simulink model "sim_elicottero"  (R2025b)
settings: Solver=VariableStepAuto  StartTime=0.0  StopTime=200  RelTol=1e-3
values from neighbouring files (symbols this model uses):
  A_nom = double(subs(A_sym_nom, [x;u], [x0;u0]))    [dataset_elicottero.m]
  aero = evalin('base','aero')    [analisi_LQG.m]
  alpha_0 = deg2rad(10)    [dataset_elicottero.m]
  B_ext_nom = [B_nom Bd_nom]    [dataset_elicottero.m]
  beta_0 = 0    [dataset_elicottero.m]
  C_angles = [ ... (first row only)    [actuator_lumped_uncertainty.m]    (also in analisi_montecarlo.m = [1 0 0 0; 0 0 1 0]; dataset_elicottero.m)
  Ddec_phys = [8.48868560985e-05  4.80771131122e-11; -3.04359895869e-06  1.06562367592e-06]    [HINF_controllers.mat]    (also in Hinf_hinfstruct.m = Du *      Ddec_scaled *      Du_inv; Hinf_synthesis_full.m = Du *      Ddec_scaled *      inv(Du))
  den_2nd = [1, 2*zeta*omega_n, omega_n^2]    [dataset_elicottero.m]
  denFalpha = [1 24.6158182311]    [HINF_controllers.mat]
  denFbeta = [1 13.1899797029]    [HINF_controllers.mat]
  F1_0 = u0_nom(1)    [dataset_elicottero.m]
  F2_0 = u0_nom(2)    [dataset_elicottero.m]
  HalphaBeta = (C_angle_meas.'*Vinv*C_angle_meas) \      (C_angle_meas.'*Vinv)    [dataset_elicottero.m]
  K_hinfsyn = minreal(          Du *          K_hinfsyn_scaled *          Dy_inv,          1e-7)    [Hinf_hinfstruct.m]    (also in Hinf_synthesis_full.m = minreal(          Du *          K_hinfsyn_scaled *          )
  K_lqg_2dof = ss(      Ac_ctrl,      Bc_ctrl,      Cc_ctrl,      Dc_ctrl)    [LQG_reg_2DOF.m]
  K_lqg_int = ss(      Ac_ctrl,      [Bcr Bcy],      Cc_ctrl,      Dc_ctrl)    [LQG_con_integratore.m]
  K_mix = minreal(          Du *          K_mix_scaled *          Dy_inv,          1e-7)    [Hinf_hinfstruct.m]    (also in Hinf_synthesis_full.m = minreal(          Du *          K_mix_scaled *          Dy_i)
  K_mu = Du * K_mu_scaled * Dy_inv    [mu_synthesis.m]
  Kalpha_tuned = pid(          alphaScaledToPhys *          Kalpha_tuned_scaled.Kp,          alphaScaledToPhys *          Kalpha_tuned_scaled.Ki,          alphaScaledToPhys *          Kalpha_tuned_scaled.Kd,          Kalpha_tuned_scaled.Tf)    [Hinf_hinfstruct.m]    (also in Hinf_synthesis_full.m = pid(          alphaScaledToPhys * Kalpha_tuned_scaled.Kp,   )
  Kbeta_tuned = pid(          betaScaledToPhys *          Kbeta_tuned_scaled.Kp,          betaScaledToPhys *          Kbeta_tuned_scaled.Ki,          betaScaledToPhys *          Kbeta_tuned_scaled.Kd,          Kbeta_tuned_scaled.Tf)    [Hinf_hinfstruct.m]    (also in Hinf_synthesis_full.m = pid(          betaScaledToPhys * Kbeta_tuned_scaled.Kp,     )
  mx_eq = cos(alpha_0) * cos(beta_0)    [dataset_elicottero.m]
  my_eq = -sin(beta_0)    [dataset_elicottero.m]
  num_2nd = omega_n^2    (= 900)    [dataset_elicottero.m]
  numFalpha = [16.7939294955 590.000844903]    [HINF_controllers.mat]
  numFbeta = [34.4835250476 9.60244651319]    [HINF_controllers.mat]
  P_nom_ext = ss(      A_nom,      B_ext_nom,      Cy,      zeros(3,4))    [dataset_elicottero.m]
  tau_d_nom = 0.02    [dataset_elicottero.m]
  umax = 5    [LQG_con_integratore.m]    (also in LQG_reg_1DOF.m; analisi_montecarlo.m = 2.5; dataset_elicottero.m)
  y_acc_eq = -p.g * sin(alpha_0)    [dataset_elicottero.m]
undefined symbols (not defined in the file or in its folder): act, sensor
libraries: simulink x20, slpidlib x2, cstblocks x2
(part 1 of 2)
settings Model: Creator=LUCA  LastModifiedBy=39345
settings DataIOCC: SaveState=on  StateSaveName=xhat_out

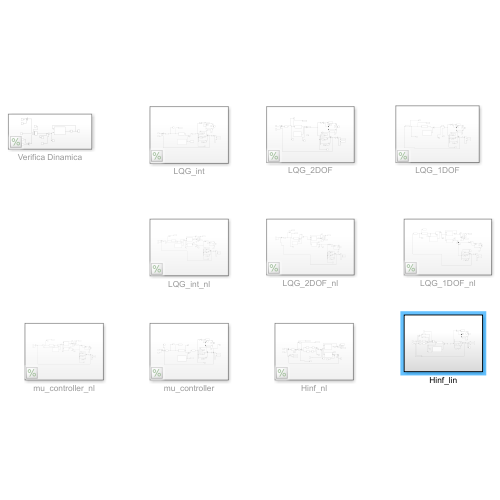
[thumbnail: Simulink's stored preview of the top-level diagram]
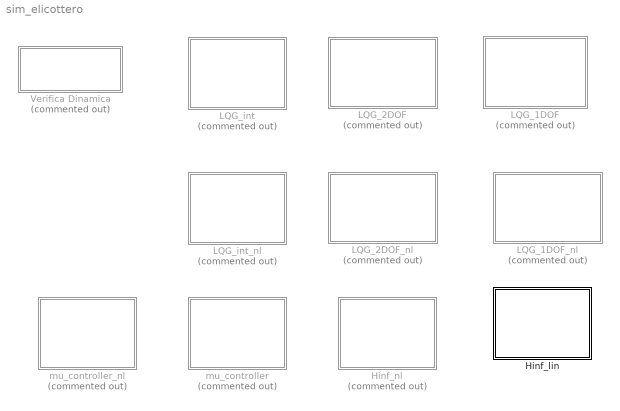
== system sim_elicottero ==
  Hinf_lin : Subsystem
  Hinf_nl : Subsystem  Commented=on
  LQG_1DOF : Subsystem  Commented=on
  LQG_1DOF_nl : Subsystem  Commented=on
  LQG_2DOF : Subsystem  Commented=on
  LQG_2DOF_nl : Subsystem  Commented=on
  LQG_int : Subsystem  Commented=on
  LQG_int_nl : Subsystem  Commented=on
  Verifica Dinamica : Subsystem  Commented=on
  mu_controller : Subsystem  Commented=on
  mu_controller_nl : Subsystem  Commented=on

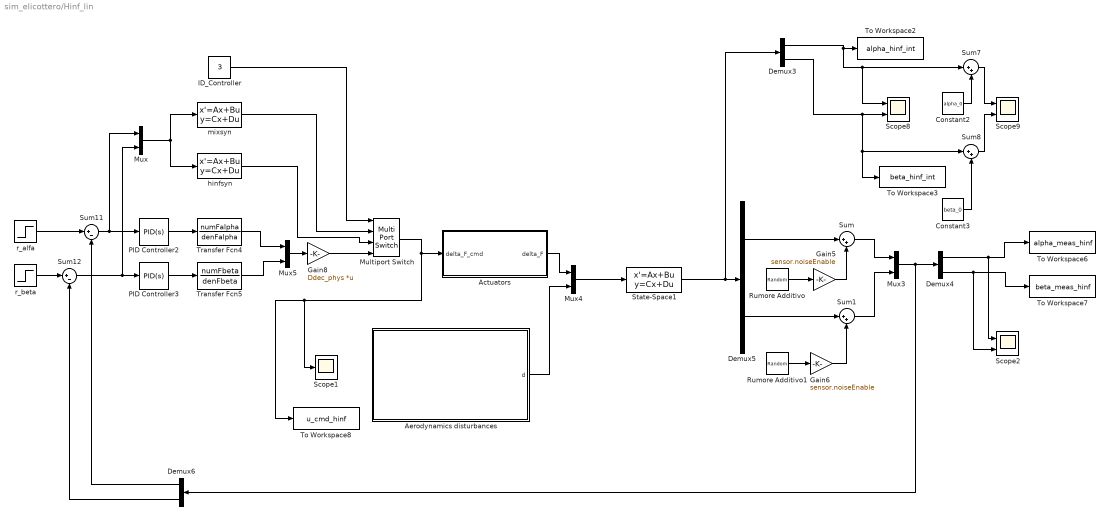
== system sim_elicottero/Hinf_lin ==
  Actuators : Subsystem
  Aerodynamics disturbances : Subsystem
  Constant2 : Constant  Value=alpha_0
  Constant3 : Constant  Value=beta_0
  Demux{3..6} (4 alike) : Demux  Outputs=2
  Gain5 : Gain  Gain=sensor.noiseEnable
  Gain6 : Gain  Gain=sensor.noiseEnable
  Gain8 : Gain  Gain=Ddec_phys  Multiplication=Matrix(K*u) (u vector)
  ID_Controller : Constant  Value=3
  Multiport Switch : MultiPortSwitch  SaturateOnIntegerOverflow=off  InputSameDT=off
  Mux{,3..5} (4 alike) : Mux  Inputs=2
  PID Controller2 : slpidlib/PID Controller  Controller=PID  Form=Parallel  TimeDomain=Continuous-time  UseExternalTs=off  SampleTime=-1  IntegratorMethod=Forward Euler  FilterMethod=Forward Euler  ControllerParametersSource=internal  P=Kalpha_tuned.Kp  I=Kalpha_tuned.Ki  UseKiTs=off  D=Kalpha_tuned.Kd  UseExternalDerivativeSource=off  N=1/Kalpha_tuned.Tf  UseFilter=on  TunerSelectOption=Transfer Function Based (PID Tuner App)  InitialConditionSource=internal  InitialConditionForIntegrator=0  InitialConditionForFilter=0  DifferentiatorICPrevScaledInput=0  ExternalReset=none  TrackingMode=off  Kt=1  LimitOutput=off  SatLimitsSource=internal  UpperSaturationLimit=inf  LowerSaturationLimit=-inf  LinearizeAsGain=on  AntiWindupMode=none  Kb=1  LimitIntegrator=off  UpperIntegratorSaturationLimit=inf  LowerIntegratorSaturationLimit=-inf  POutMin=[]  POutMax=[]  IOutMin=[]  IOutMax=[]  DOutMin=[]  DOutMax=[]  NOutMin=[]  NOutMax=[]  SumOutMin=[]  SumOutMax=[]  SaturationOutMin=[]  SaturationOutMax=[]  PParamMin=[]  PParamMax=[]  IParamMin=[]  IParamMax=[]  DParamMin=[]  DParamMax=[]  NParamMin=[]  NParamMax=[]  KbParamMin=[]  KbParamMax=[]  KtParamMin=[]  KtParamMax=[]  KbOutMin=[]  KbOutMax=[]  KtOutMin=[]  KtOutMax=[]  IntegratorOutMin=[]  IntegratorOutMax=[]  FilterOutMin=[]  FilterOutMax=[]  SumI1OutMin=[]  SumI1OutMax=[]  SumI2OutMin=[]  SumI2OutMax=[]  SumI3OutMin=[]  SumI3OutMax=[]  SumI4OutMin=[]  SumI4OutMax=[]  SumDOutMin=[]  SumDOutMax=[]  DifferentiatorOutMin=[]  DifferentiatorOutMax=[]  FilterDiffOutCoefMin=[]  FilterDiffOutCoefMax=[]  ReciprocalOutMin=[]  ReciprocalOutMax=[]  SumDenOutMin=[]  SumDenOutMax=[]  SumNumOutMin=[]  SumNumOutMax=[]  DivideOutMin=[]  DivideOutMax=[]  UdiffTsProdOutMin=[]  UdiffTsProdOutMax=[]  NTsProdOutMin=[]  NTsProdOutMax=[]  UintegralTsProdOutMin=[]  UintegralTsProdOutMax=[]  UngainTsProdOutMin=[]  UngainTsProdOutMax=[]  ClampingZeroOutDataTypeStr=Inherit: Inherit via back propagation  ClampingZeroOutMin=[]  ClampingZeroOutMax=[]  FilterDenConstantOutDataTypeStr=Inherit: Inherit via back propagation  FilterDenConstantOutMin=[]  FilterDenConstantOutMax=[]  PCopyOutDataTypeStr=Inherit: Inherit via back propagation  PCopyOutMin=[]  PCopyOutMax=[]  NCopyOutDataTypeStr=Inherit: Inherit via back propagation  NCopyOutMin=[]  NCopyOutMax=[]  IntegratorContinuousStateAttributes=''  IntegratorStateMustResolveToSignalObject=off  IntegratorRTWStateStorageClass=Auto  FilterContinuousStateAttributes=''  FilterStateMustResolveToSignalObject=off  FilterRTWStateStorageClass=Auto  ParallelPVariant=InternalParameters  IdealPVariant=Disabled  IVariant=InternalParameters  DVariant=InternalParameters  IntegratorVariant=Continuous  SatVariant=Disabled  AWVariant=Passthrough  PCopyVariant=Disabled  TRVariant=Disabled  FdbkBlocksVariant=Forward  IdealPFdbkVariant=Disabled  SatFdbkVariant=Disabled  DerivativeFilterVariant=ContFilter  NVariant=InternalParameters  NCopyVariant=Disabled  FilterICVariant=InternalICsFilter  IntegratorICVariant=InternalICs  ExternalResetVariant=Disabled  TRSumVariant=Passthrough  SumFdbkVariant=Disabled  SumVariant=Sum_PID  TsampFilterVariant=InternalTs  TsampNgainVariant=Passthrough  TsampIntegralVariant=Disabled_SignalSpec  ExternalSaturationOutDataTypeStr=Inherit: Same as second input  DerivativeSourceVariant=ErrorSignal  PreIntVariant=InternalPreInt
  PID Controller3 : slpidlib/PID Controller  Controller=PID  Form=Parallel  TimeDomain=Continuous-time  UseExternalTs=off  SampleTime=-1  IntegratorMethod=Forward Euler  FilterMethod=Forward Euler  ControllerParametersSource=internal  P=Kbeta_tuned.Kp  I=Kbeta_tuned.Ki  UseKiTs=off  D=Kbeta_tuned.Kd  UseExternalDerivativeSource=off  N=1/Kbeta_tuned.tf  UseFilter=on  TunerSelectOption=Transfer Function Based (PID Tuner App)  InitialConditionSource=internal  InitialConditionForIntegrator=0  InitialConditionForFilter=0  DifferentiatorICPrevScaledInput=0  ExternalReset=none  TrackingMode=off  Kt=1  LimitOutput=off  SatLimitsSource=internal  UpperSaturationLimit=inf  LowerSaturationLimit=-inf  LinearizeAsGain=on  AntiWindupMode=none  Kb=1  LimitIntegrator=off  UpperIntegratorSaturationLimit=inf  LowerIntegratorSaturationLimit=-inf  POutMin=[]  POutMax=[]  IOutMin=[]  IOutMax=[]  DOutMin=[]  DOutMax=[]  NOutMin=[]  NOutMax=[]  SumOutMin=[]  SumOutMax=[]  SaturationOutMin=[]  SaturationOutMax=[]  PParamMin=[]  PParamMax=[]  IParamMin=[]  IParamMax=[]  DParamMin=[]  DParamMax=[]  NParamMin=[]  NParamMax=[]  KbParamMin=[]  KbParamMax=[]  KtParamMin=[]  KtParamMax=[]  KbOutMin=[]  KbOutMax=[]  KtOutMin=[]  KtOutMax=[]  IntegratorOutMin=[]  IntegratorOutMax=[]  FilterOutMin=[]  FilterOutMax=[]  SumI1OutMin=[]  SumI1OutMax=[]  SumI2OutMin=[]  SumI2OutMax=[]  SumI3OutMin=[]  SumI3OutMax=[]  SumI4OutMin=[]  SumI4OutMax=[]  SumDOutMin=[]  SumDOutMax=[]  DifferentiatorOutMin=[]  DifferentiatorOutMax=[]  FilterDiffOutCoefMin=[]  FilterDiffOutCoefMax=[]  ReciprocalOutMin=[]  ReciprocalOutMax=[]  SumDenOutMin=[]  SumDenOutMax=[]  SumNumOutMin=[]  SumNumOutMax=[]  DivideOutMin=[]  DivideOutMax=[]  UdiffTsProdOutMin=[]  UdiffTsProdOutMax=[]  NTsProdOutMin=[]  NTsProdOutMax=[]  UintegralTsProdOutMin=[]  UintegralTsProdOutMax=[]  UngainTsProdOutMin=[]  UngainTsProdOutMax=[]  ClampingZeroOutDataTypeStr=Inherit: Inherit via back propagation  ClampingZeroOutMin=[]  ClampingZeroOutMax=[]  FilterDenConstantOutDataTypeStr=Inherit: Inherit via back propagation  FilterDenConstantOutMin=[]  FilterDenConstantOutMax=[]  PCopyOutDataTypeStr=Inherit: Inherit via back propagation  PCopyOutMin=[]  PCopyOutMax=[]  NCopyOutDataTypeStr=Inherit: Inherit via back propagation  NCopyOutMin=[]  NCopyOutMax=[]  IntegratorContinuousStateAttributes=''  IntegratorStateMustResolveToSignalObject=off  IntegratorRTWStateStorageClass=Auto  FilterContinuousStateAttributes=''  FilterStateMustResolveToSignalObject=off  FilterRTWStateStorageClass=Auto  ParallelPVariant=InternalParameters  IdealPVariant=Disabled  IVariant=InternalParameters  DVariant=InternalParameters  IntegratorVariant=Continuous  SatVariant=Disabled  AWVariant=Passthrough  PCopyVariant=Disabled  TRVariant=Disabled  FdbkBlocksVariant=Forward  IdealPFdbkVariant=Disabled  SatFdbkVariant=Disabled  DerivativeFilterVariant=ContFilter  NVariant=InternalParameters  NCopyVariant=Disabled  FilterICVariant=InternalICsFilter  IntegratorICVariant=InternalICs  ExternalResetVariant=Disabled  TRSumVariant=Passthrough  SumFdbkVariant=Disabled  SumVariant=Sum_PID  TsampFilterVariant=InternalTs  TsampNgainVariant=Passthrough  TsampIntegralVariant=Disabled_SignalSpec  ExternalSaturationOutDataTypeStr=Inherit: Same as second input  DerivativeSourceVariant=ErrorSignal  PreIntVariant=InternalPreInt
  Rumore Additivo : RandomNumber  Variance=sensor.acc.var  Seed=sensor.seed  SampleTime=sensor.acc.Ts
  Rumore Additivo1 : RandomNumber  Variance=sensor.mag.var  Seed=sensor.seed+1  SampleTime=sensor.mag.Ts
  Scope1 : Scope
      settings: ActiveDisplayYMinimum=-1  ActiveDisplayYMaximum=1  DataLoggingVariableName=ScopeData23
  Scope2 : Scope  NumInputPorts=2
      settings: ActiveDisplayYMinimum=-0.051852365293432415  ActiveDisplayYMaximum=0.26472523909457119  DataLoggingVariableName=ScopeData46
  Scope8 : Scope  NumInputPorts=2
      settings: ActiveDisplayYMinimum=-0.063740224539216614  ActiveDisplayYMaximum=0.371715972306629  DataLoggingVariableName=ScopeData40
  Scope9 : Scope  NumInputPorts=2
      settings: ActiveDisplayYMinimum=-0.5568080690889109  ActiveDisplayYMaximum=1.993995872875248  DataLoggingVariableName=ScopeData41
  State-Space1 : StateSpace  A=A_nom  B=B_ext_nom  C=C_angles  D=zeros(2,4)  InitialCondition=0
  Sum{,1,7..8} (4 alike) : Sum  Inputs=|++
  Sum11 : Sum  Inputs=|+-
  Sum12 : Sum  Inputs=|+-
  To Workspace2 : ToWorkspace  VariableName=alpha_hinf_int  SaveFormat=Timeseries  SampleTime=-1
  To Workspace3 : ToWorkspace  VariableName=beta_hinf_int  SaveFormat=Timeseries  SampleTime=-1
  To Workspace6 : ToWorkspace  VariableName=alpha_meas_hinf  SaveFormat=Timeseries  SampleTime=-1
  To Workspace7 : ToWorkspace  VariableName=beta_meas_hinf  SaveFormat=Timeseries  SampleTime=-1
  To Workspace8 : ToWorkspace  VariableName=u_cmd_hinf  SaveFormat=Timeseries  SampleTime=-1
  Transfer Fcn4 : TransferFcn  Numerator=numFalpha  Denominator=denFalpha
  Transfer Fcn5 : TransferFcn  Numerator=numFbeta  Denominator=denFbeta
  hinfsyn : StateSpace  A=K_hinfsyn.A  B=K_hinfsyn.B  C=K_hinfsyn.C  D=K_hinfsyn.D  InitialCondition=0
  mixsyn : StateSpace  A=K_mix.A  B=K_mix.B  C=K_mix.C  D=K_mix.D  InitialCondition=0
  r_alfa : Step  After=deg2rad(3)  SampleTime=0
  r_beta : Step  After=0  SampleTime=0
  wires:
  Gain5/1 -> Sum/2
  Constant3/1 -> Sum8/2
  Rumore Additivo/1 -> Gain5/1
  Sum8/1 -> Scope9/2
  Mux3/1 -> Demux6/1, Demux4/1
  Gain6/1 -> Sum1/2
  Demux3/1 -> Sum7/1, Scope8/1, To Workspace2/1
  Actuators/1(delta_F) -> Mux4/1
  Demux4/1 -> Scope2/1, To Workspace6/1
  Rumore Additivo1/1 -> Gain6/1
  Constant2/1 -> Sum7/2
  Aerodynamics disturbances/1(d) -> Mux4/2
  State-Space1/1 -> Demux5/1, Demux3/1
  Sum7/1 -> Scope9/1
  Demux3/2 -> Sum8/1, To Workspace3/1, Scope8/2
  Demux6/2 -> Sum12/2
  Demux6/1 -> Sum11/2
  r_alfa/1 -> Sum11/1
  r_beta/1 -> Sum12/1
  Transfer Fcn4/1 -> Mux5/1
  PID Controller2/1 -> Transfer Fcn4/1
  Sum12/1 -> PID Controller3/1, Mux/2
  Gain8/1 -> Multiport Switch/4
  PID Controller3/1 -> Transfer Fcn5/1
  Mux5/1 -> Gain8/1
  Demux5/2 -> Sum1/1
  Sum1/1 -> Mux3/2
  Demux5/1 -> Sum/1
  Sum/1 -> Mux3/1
  Transfer Fcn5/1 -> Mux5/2
  Sum11/1 -> PID Controller2/1, Mux/1
  Mux/1 -> hinfsyn/1, mixsyn/1
  mixsyn/1 -> Multiport Switch/2
  hinfsyn/1 -> Multiport Switch/3
  ID_Controller/1 -> Multiport Switch/1
  Multiport Switch/1 -> To Workspace8/1, Scope1/1, Actuators/1(delta_F_cmd)
  Mux4/1 -> State-Space1/1
  Demux4/2 -> Scope2/2, To Workspace7/1

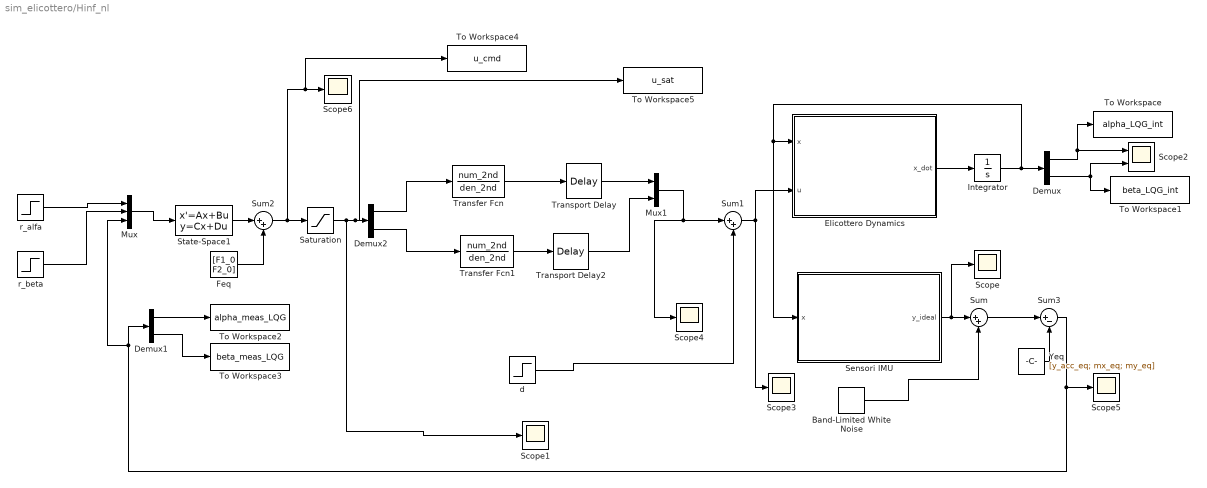
== system sim_elicottero/Hinf_nl ==
  Band-Limited White Noise : simulink/Sources/Band-Limited White Noise  Cov=[1e-3, 1e-3, 1e-3]  Ts=0.01  seed=[23341 23342 23343]
  Demux : Demux  Outputs=2
  Demux1 : Demux  Outputs=2
  Demux2 : Demux  Outputs=2
  Elicottero Dynamics : MATLAB Function  TreatAsAtomicUnit=on
  Feq : Constant  Value=[F1_0 F2_0]
  Integrator : Integrator
  Mux : Mux  Inputs=3
  Mux1 : Mux  Inputs=2
  Saturation : Saturate  UpperLimit=umax  LowerLimit=-umax
  Scope{,1,3..6} (6 alike) : Scope
      Scope settings: ActiveDisplayYMinimum=-1.6240661630355766  ActiveDisplayYMaximum=0.25200758348707814  DataLoggingVariableName=ScopeData14
      Scope1 settings: ActiveDisplayYMinimum=-3.9672250570633585  ActiveDisplayYMaximum=4.5871365678108127  DataLoggingVariableName=ScopeData15
      Scope3 settings: ActiveDisplayYMinimum=-0.066808898460173932  ActiveDisplayYMaximum=0.16260152032849579  DataLoggingVariableName=ScopeData17
      Scope4 settings: ActiveDisplayYMinimum=-0.20524936057198231  ActiveDisplayYMaximum=0.3898908376036152  DataLoggingVariableName=ScopeData18
      Scope5 settings: DataLoggingVariableName=ScopeData20
      Scope6 settings: ActiveDisplayYMinimum=-1  ActiveDisplayYMaximum=1  DataLoggingVariableName=ScopeData19
  Scope2 : Scope  NumInputPorts=2
      settings: ActiveDisplayYMinimum=-0.12109022574417846  ActiveDisplayYMaximum=0.4458099433494796  DataLoggingVariableName=ScopeData16
  Sensori IMU : MATLAB Function  TreatAsAtomicUnit=on
  State-Space1 : StateSpace  A=K_lqg_int.A  B=K_lqg_int.B  C=K_lqg_int.C  D=K_lqg_int.D  InitialCondition=0  ContinuousStateAttributes='stati_stimati'
  Sum : Sum  Inputs=|++
  Sum1 : Sum  Inputs=|++
  Sum2 : Sum  Inputs=|++
  Sum3 : Sum  Inputs=|+-
  To Workspace : ToWorkspace  VariableName=alpha_LQG_int  SaveFormat=Timeseries  SampleTime=-1
  To Workspace1 : ToWorkspace  VariableName=beta_LQG_int  SaveFormat=Timeseries  SampleTime=-1
  To Workspace2 : ToWorkspace  VariableName=alpha_meas_LQG  SaveFormat=Timeseries  SampleTime=-1
  To Workspace3 : ToWorkspace  VariableName=beta_meas_LQG  SaveFormat=Timeseries  SampleTime=-1
  To Workspace4 : ToWorkspace  VariableName=u_cmd  SaveFormat=Timeseries  SampleTime=-1
  To Workspace5 : ToWorkspace  VariableName=u_sat  SaveFormat=Timeseries  SampleTime=-1
  Transfer Fcn : TransferFcn  Numerator=num_2nd  Denominator=den_2nd
  Transfer Fcn1 : TransferFcn  Numerator=num_2nd  Denominator=den_2nd
  Transport Delay : TransportDelay  DelayTime=tau_d_nom
  Transport Delay2 : TransportDelay  DelayTime=tau_d_nom
  Yeq : Constant  Value=[y_acc_eq; mx_eq; my_eq]
  d : Step  Time=10  After=0.05  SampleTime=0
  r_alfa : Step  After=0.1  SampleTime=0
  r_beta : Step  After=0  SampleTime=0
  wires:
  Mux1/1 -> Sum1/1, Scope4/1
  r_alfa/1 -> Mux/1
  Saturation/1 -> To Workspace5/1, Demux2/1, Scope1/1
  Sum1/1 -> Elicottero Dynamics/2(u), Scope3/1
  Mux/1 -> State-Space1/1
  Sensori IMU/1(y_ideal) -> Scope/1, Sum/1
  d/1 -> Sum1/2
  Band-Limited White Noise/1 -> Sum/2
  Demux2/2 -> Transfer Fcn1/1
  Demux2/1 -> Transfer Fcn/1
  Transfer Fcn1/1 -> Transport Delay2/1
  Transport Delay2/1 -> Mux1/2
  Transfer Fcn/1 -> Transport Delay/1
  Transport Delay/1 -> Mux1/1
  Demux1/1 -> To Workspace2/1
  Demux1/2 -> To Workspace3/1
  r_beta/1 -> Mux/2
  Demux/1 -> To Workspace/1, Scope2/1
  Demux/2 -> Scope2/2, To Workspace1/1
  Elicottero Dynamics/1(x_dot) -> Integrator/1
  Integrator/1 -> Sensori IMU/1(x), Elicottero Dynamics/1(x), Demux/1
  State-Space1/1 -> Sum2/1
  Feq/1 -> Sum2/2
  Sum2/1 -> To Workspace4/1, Scope6/1, Saturation/1
  Sum/1 -> Sum3/1
  Yeq/1 -> Sum3/2
  Sum3/1 -> Scope5/1, Demux1/1, Mux/3

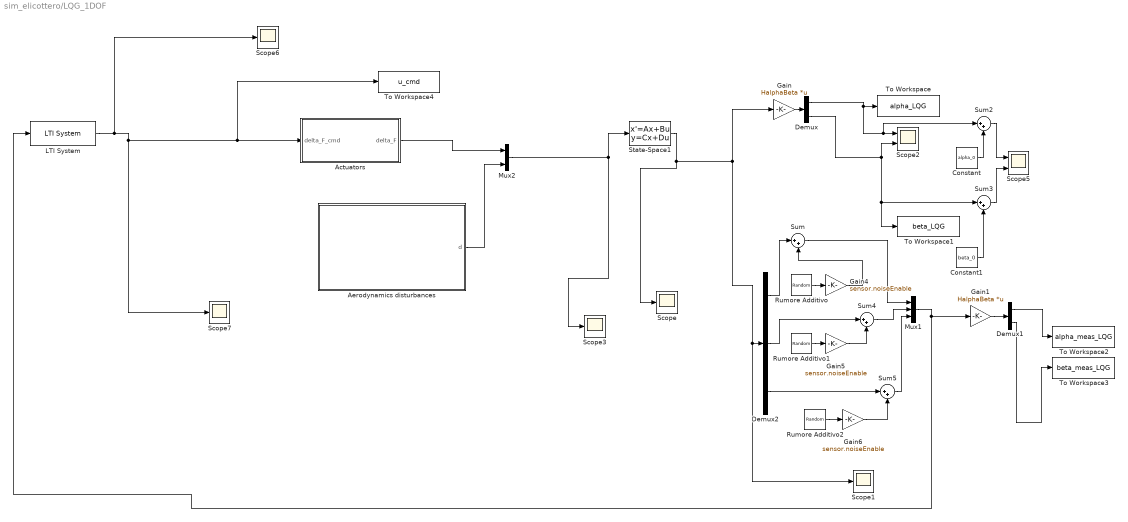
== system sim_elicottero/LQG_1DOF ==
  Actuators : Subsystem
  Aerodynamics disturbances : Subsystem
  Constant : Constant  Value=alpha_0
  Constant1 : Constant  Value=beta_0
  Demux : Demux  Outputs=2
  Demux1 : Demux  Outputs=2
  Demux2 : Demux  Outputs=3
  Gain : Gain  Gain=HalphaBeta  Multiplication=Matrix(K*u)
  Gain1 : Gain  Gain=HalphaBeta  Multiplication=Matrix(K*u)
  Gain4 : Gain  Gain=sensor.noiseEnable
  Gain5 : Gain  Gain=sensor.noiseEnable
  Gain6 : Gain  Gain=sensor.noiseEnable
  LTI System : cstblocks/LTI System  sys=K_lqg_reg  IC=[]  PadeOrder=0
  Mux1 : Mux  Inputs=3
  Mux2 : Mux  Inputs=2
  Rumore Additivo : RandomNumber  Variance=sensor.acc.var  Seed=sensor.seed  SampleTime=sensor.acc.Ts
  Rumore Additivo1 : RandomNumber  Variance=sensor.mag.var  Seed=sensor.seed+1  SampleTime=sensor.mag.Ts
  Rumore Additivo2 : RandomNumber  Variance=sensor.mag.var  Seed=sensor.seed+2  SampleTime=sensor.mag.Ts
  Scope{,1,3,6..7} (5 alike) : Scope
      Scope settings: ActiveDisplayYMinimum=-0.098672452572545172  ActiveDisplayYMaximum=0.25214523323110316  DataLoggingVariableName=ScopeData5
      Scope1 settings: ActiveDisplayYMinimum=-1.6240661630355766  ActiveDisplayYMaximum=0.25200758348707814  DataLoggingVariableName=ScopeData8
      Scope3 settings: ActiveDisplayYMinimum=-0.066808898460173932  ActiveDisplayYMaximum=0.16260152032849579  DataLoggingVariableName=ScopeData10
      Scope6 settings: ActiveDisplayYMinimum=-1  ActiveDisplayYMaximum=1  DataLoggingVariableName=ScopeData12
      Scope7 settings: ActiveDisplayYMinimum=-1  ActiveDisplayYMaximum=1  DataLoggingVariableName=ScopeData13
  Scope2 : Scope  NumInputPorts=2
      settings: ActiveDisplayYMinimum=-0.039158982680938585  ActiveDisplayYMaximum=0.10762825192016658  DataLoggingVariableName=ScopeData9
  Scope5 : Scope  NumInputPorts=2
      settings: ActiveDisplayYMinimum=-0.056599950333026186  ActiveDisplayYMaximum=0.28073891791993266  DataLoggingVariableName=ScopeData11
  State-Space1 : StateSpace  A=P_nom_ext.A  B=P_nom_ext.B  C=P_nom_ext.C  D=P_nom_ext.D  InitialCondition=0
  Sum{,2..5} (5 alike) : Sum  Inputs=|++
  To Workspace : ToWorkspace  VariableName=alpha_LQG  SaveFormat=Timeseries  SampleTime=-1
  To Workspace1 : ToWorkspace  VariableName=beta_LQG  SaveFormat=Timeseries  SampleTime=-1
  To Workspace2 : ToWorkspace  VariableName=alpha_meas_LQG  SaveFormat=Timeseries  SampleTime=-1
  To Workspace3 : ToWorkspace  VariableName=beta_meas_LQG  SaveFormat=Timeseries  SampleTime=-1
  To Workspace4 : ToWorkspace  VariableName=u_cmd  SaveFormat=Timeseries  SampleTime=-1
  wires:
  LTI System/1 -> To Workspace4/1, Actuators/1(delta_F_cmd), Scope7/1, Scope6/1
  Mux2/1 -> State-Space1/1, Scope3/1
  Aerodynamics disturbances/1(d) -> Mux2/2
  Actuators/1(delta_F) -> Mux2/1
  Demux2/2 -> Sum4/1
  Gain4/1 -> Sum/2
  Demux/2 -> Sum3/1, To Workspace1/1, Scope2/2
  Sum/1 -> Mux1/1
  State-Space1/1 -> Demux2/1, Scope1/1, Gain/1, Scope/1
  Rumore Additivo2/1 -> Gain6/1
  Sum5/1 -> Mux1/3
  Demux/1 -> Sum2/1, Scope2/1, To Workspace/1
  Demux1/2 -> To Workspace3/1
  Rumore Additivo/1 -> Gain4/1
  Constant/1 -> Sum2/2
  Sum2/1 -> Scope5/1
  Demux2/3 -> Sum5/1
  Sum4/1 -> Mux1/2
  Rumore Additivo1/1 -> Gain5/1
  Gain/1 -> Demux/1
  Constant1/1 -> Sum3/2
  Gain1/1 -> Demux1/1
  Demux2/1 -> Sum/1
  Gain5/1 -> Sum4/2
  Mux1/1 -> LTI System/1, Gain1/1
  Sum3/1 -> Scope5/2
  Demux1/1 -> To Workspace2/1
  Gain6/1 -> Sum5/2

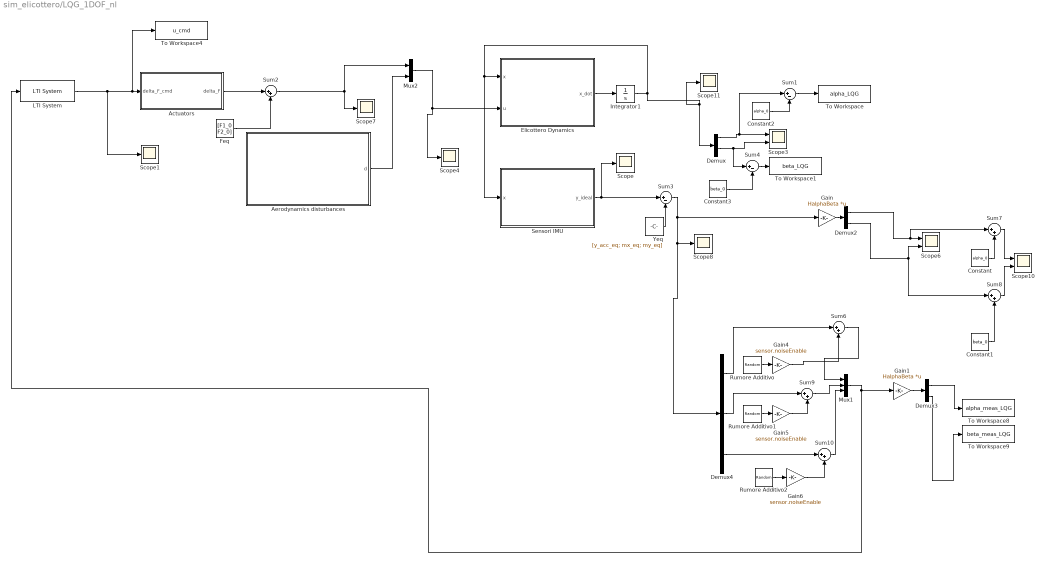
== system sim_elicottero/LQG_1DOF_nl ==
  Actuators : Subsystem
  Aerodynamics disturbances : Subsystem
  Constant : Constant  Value=alpha_0
  Constant1 : Constant  Value=beta_0
  Constant2 : Constant  Value=alpha_0
  Constant3 : Constant  Value=beta_0
  Demux : Demux
  Demux2 : Demux  Outputs=2
  Demux3 : Demux  Outputs=2
  Demux4 : Demux  Outputs=3
  Elicottero Dynamics : MATLAB Function  TreatAsAtomicUnit=on
  Feq : Constant  Value=[F1_0 F2_0]
  Gain : Gain  Gain=HalphaBeta  Multiplication=Matrix(K*u)
  Gain1 : Gain  Gain=HalphaBeta  Multiplication=Matrix(K*u)
  Gain4 : Gain  Gain=sensor.noiseEnable
  Gain5 : Gain  Gain=sensor.noiseEnable
  Gain6 : Gain  Gain=sensor.noiseEnable
  Integrator1 : Integrator  InitialCondition=[alpha_0; 0; beta_0; 0]
  LTI System : cstblocks/LTI System  sys=K_lqg_reg  IC=[]  PadeOrder=0
  Mux1 : Mux  Inputs=3
  Mux2 : Mux  Inputs=2
  Rumore Additivo : RandomNumber  Variance=sensor.acc.var  Seed=sensor.seed  SampleTime=sensor.acc.Ts
  Rumore Additivo1 : RandomNumber  Variance=sensor.mag.var  Seed=sensor.seed+1  SampleTime=sensor.mag.Ts
  Rumore Additivo2 : RandomNumber  Variance=sensor.mag.var  Seed=sensor.seed+2  SampleTime=sensor.mag.Ts
  Scope{,1,4,7..8,11} (6 alike) : Scope
      Scope settings: ActiveDisplayYMinimum=-1.6240661630355766  ActiveDisplayYMaximum=0.25200758348707814  DataLoggingVariableName=ScopeData22
      Scope1 settings: ActiveDisplayYMinimum=-0.85201275058268955  ActiveDisplayYMaximum=3.9243929593456111
      Scope11 settings: ActiveDisplayYMinimum=-0.054376475161351162  ActiveDisplayYMaximum=0.224772679209085  DataLoggingVariableName=ScopeData35
      Scope4 settings: ActiveDisplayYMinimum=-0.11442663629112786  ActiveDisplayYMaximum=0.10867739086166754  DataLoggingVariableName=ScopeData4
      Scope7 settings: ActiveDisplayYMinimum=-0.16116164249761136  ActiveDisplayYMaximum=0.54820504636646727  DataLoggingVariableName=ScopeData33
      Scope8 settings: DataLoggingVariableName=ScopeData25
  Scope10 : Scope  NumInputPorts=2
      settings: ActiveDisplayYMinimum=-0.054885502995600327  ActiveDisplayYMaximum=0.26421908209196954  DataLoggingVariableName=ScopeData34
  Scope3 : Scope  NumInputPorts=2
      settings: ActiveDisplayYMinimum=-0.056861495742625029  ActiveDisplayYMaximum=0.28133520253821959  DataLoggingVariableName=ScopeData37
  Scope6 : Scope  NumInputPorts=2
      settings: ActiveDisplayYMinimum=-0.033068887345671219  ActiveDisplayYMaximum=0.0678695412426075  DataLoggingVariableName=ScopeData38
  Sensori IMU : MATLAB Function  TreatAsAtomicUnit=on
  Sum1 : Sum  Inputs=|+-
  Sum{2,6..10} (6 alike) : Sum  Inputs=|++
  Sum3 : Sum  Inputs=|+-
  Sum4 : Sum  Inputs=|+-
  To Workspace : ToWorkspace  VariableName=alpha_LQG  SaveFormat=Timeseries  SampleTime=-1
  To Workspace1 : ToWorkspace  VariableName=beta_LQG  SaveFormat=Timeseries  SampleTime=-1
  To Workspace4 : ToWorkspace  VariableName=u_cmd  SaveFormat=Timeseries  SampleTime=-1
  To Workspace8 : ToWorkspace  VariableName=alpha_meas_LQG  SaveFormat=Timeseries  SampleTime=-1
  To Workspace9 : ToWorkspace  VariableName=beta_meas_LQG  SaveFormat=Timeseries  SampleTime=-1
  Yeq : Constant  Value=[y_acc_eq; mx_eq; my_eq]
  wires:
  Yeq/1 -> Sum3/2
  Sum3/1 -> Demux4/1, Scope8/1, Gain/1
  Sensori IMU/1(y_ideal) -> Sum3/1, Scope/1
  Feq/1 -> Sum2/2
  LTI System/1 -> Scope1/1, To Workspace4/1, Actuators/1(delta_F_cmd)
  Actuators/1(delta_F) -> Sum2/1
  Sum2/1 -> Scope7/1, Mux2/1
  Mux2/1 -> Scope4/1, Elicottero Dynamics/2(u)
  Aerodynamics disturbances/1(d) -> Mux2/2
  Demux/3 -> Sum4/1, Scope3/2
  Sum10/1 -> Mux1/3
  Sum7/1 -> Scope10/1
  Demux4/2 -> Sum9/1
  Gain4/1 -> Sum6/2
  Gain6/1 -> Sum10/2
  Sum6/1 -> Mux1/1
  Demux2/2 -> Sum8/1, Scope6/2
  Demux4/3 -> Sum10/1
  Sum4/1 -> To Workspace1/1
  Constant1/1 -> Sum8/2
  Demux3/1 -> To Workspace8/1
  Demux2/1 -> Sum7/1, Scope6/1
  Constant/1 -> Sum7/2
  Rumore Additivo/1 -> Gain4/1
  Demux4/1 -> Sum6/1
  Sum1/1 -> To Workspace/1
  Sum9/1 -> Mux1/2
  Mux1/1 -> LTI System/1, Gain1/1
  Demux3/2 -> To Workspace9/1
  Constant3/1 -> Sum4/2
  Sum8/1 -> Scope10/2
  Constant2/1 -> Sum1/2
  Rumore Additivo1/1 -> Gain5/1
  Gain/1 -> Demux2/1
  Gain1/1 -> Demux3/1
  Integrator1/1 -> Demux/1, Scope11/1, Sensori IMU/1(x), Elicottero Dynamics/1(x)
  Demux/1 -> Sum1/1, Scope3/1
  Rumore Additivo2/1 -> Gain6/1
  Gain5/1 -> Sum9/2
  Elicottero Dynamics/1(x_dot) -> Integrator1/1

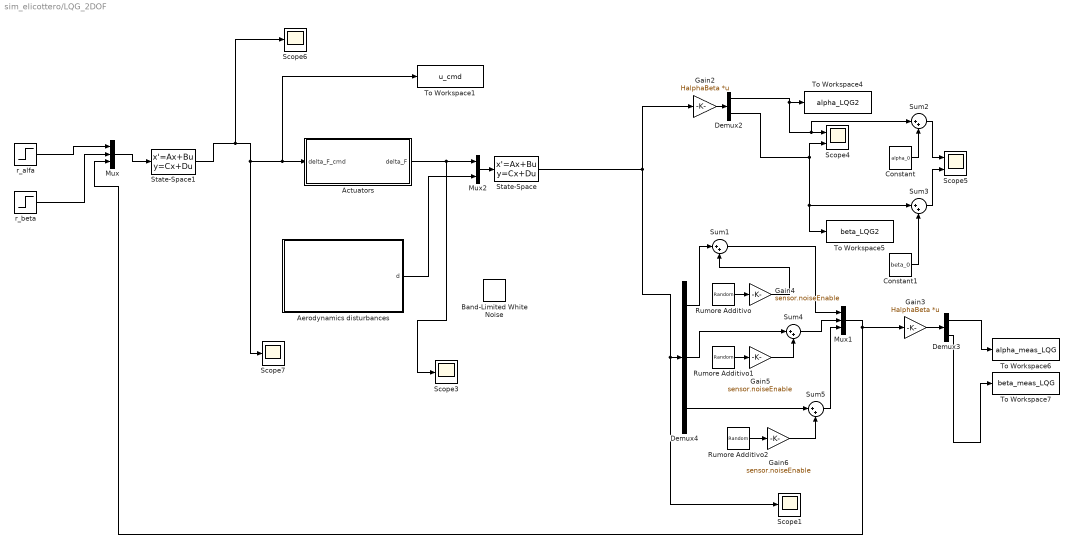
== system sim_elicottero/LQG_2DOF ==
  Actuators : Subsystem
  Aerodynamics disturbances : Subsystem
  Band-Limited White Noise : simulink/Sources/Band-Limited White Noise  Cov=[1e-3, 1e-3]  Ts=0.01  seed=[23341, 23342]
  Constant : Constant  Value=alpha_0
  Constant1 : Constant  Value=beta_0
  Demux2 : Demux  Outputs=2
  Demux3 : Demux  Outputs=2
  Demux4 : Demux  Outputs=3
  Gain2 : Gain  Gain=HalphaBeta  Multiplication=Matrix(K*u)
  Gain3 : Gain  Gain=HalphaBeta  Multiplication=Matrix(K*u)
  Gain4 : Gain  Gain=sensor.noiseEnable
  Gain5 : Gain  Gain=sensor.noiseEnable
  Gain6 : Gain  Gain=sensor.noiseEnable
  Mux : Mux  Inputs=3
  Mux1 : Mux  Inputs=3
  Mux2 : Mux  Inputs=2
  Rumore Additivo : RandomNumber  Variance=sensor.acc.var  Seed=sensor.seed  SampleTime=sensor.acc.Ts
  Rumore Additivo1 : RandomNumber  Variance=sensor.mag.var  Seed=sensor.seed+1  SampleTime=sensor.mag.Ts
  Rumore Additivo2 : RandomNumber  Variance=sensor.mag.var  Seed=sensor.seed+2  SampleTime=sensor.mag.Ts
  Scope{1,3,6..7} (4 alike) : Scope
      Scope1 settings: ActiveDisplayYMinimum=-1.6240661630355766  ActiveDisplayYMaximum=0.25200758348707814  DataLoggingVariableName=ScopeData29
      Scope3 settings: ActiveDisplayYMinimum=-0.066808898460173932  ActiveDisplayYMaximum=0.16260152032849579  DataLoggingVariableName=ScopeData3
      Scope6 settings: ActiveDisplayYMinimum=-1  ActiveDisplayYMaximum=1  DataLoggingVariableName=ScopeData6
      Scope7 settings: ActiveDisplayYMinimum=-1  ActiveDisplayYMaximum=1  DataLoggingVariableName=ScopeData7
  Scope4 : Scope  NumInputPorts=2
      settings: ActiveDisplayYMinimum=-0.038542260634245373  ActiveDisplayYMaximum=0.1098096362913842  DataLoggingVariableName=ScopeData30
  Scope5 : Scope  NumInputPorts=2
      settings: ActiveDisplayYMinimum=-0.044660276074974345  ActiveDisplayYMaximum=0.28398980869776269  DataLoggingVariableName=ScopeData31
  State-Space : StateSpace  A=P_nom_ext.A  B=P_nom_ext.B  C=P_nom_ext.C  D=P_nom_ext.D  InitialCondition=0
  State-Space1 : StateSpace  A=K_lqg_2dof.A  B=K_lqg_2dof.B  C=K_lqg_2dof.C  D=K_lqg_2dof.D  InitialCondition=0  ContinuousStateAttributes='stati_stimati'
  Sum{1..5} (5 alike) : Sum  Inputs=|++
  To Workspace1 : ToWorkspace  VariableName=u_cmd  SaveFormat=Timeseries  SampleTime=-1
  To Workspace4 : ToWorkspace  VariableName=alpha_LQG2  SaveFormat=Timeseries  SampleTime=-1
  To Workspace5 : ToWorkspace  VariableName=beta_LQG2  SaveFormat=Timeseries  SampleTime=-1
  To Workspace6 : ToWorkspace  VariableName=alpha_meas_LQG  SaveFormat=Timeseries  SampleTime=-1
  To Workspace7 : ToWorkspace  VariableName=beta_meas_LQG  SaveFormat=Timeseries  SampleTime=-1
  r_alfa : Step  After=deg2rad(3)  SampleTime=0
  r_beta : Step  After=0  SampleTime=0
  wires:
  State-Space1/1 -> To Workspace1/1, Actuators/1(delta_F_cmd), Scope7/1, Scope6/1
  Mux/1 -> State-Space1/1
  Mux2/1 -> State-Space/1
  Aerodynamics disturbances/1(d) -> Mux2/2
  Sum3/1 -> Scope5/2
  Sum5/1 -> Mux1/3
  Gain6/1 -> Sum5/2
  Demux3/1 -> To Workspace6/1
  Rumore Additivo1/1 -> Gain5/1
  Gain4/1 -> Sum1/2
  Gain3/1 -> Demux3/1
  Constant1/1 -> Sum3/2
  Sum4/1 -> Mux1/2
  Demux2/1 -> Sum2/1, Scope4/1, To Workspace4/1
  Gain2/1 -> Demux2/1
  State-Space/1 -> Demux4/1, Scope1/1, Gain2/1
  Rumore Additivo2/1 -> Gain6/1
  Gain5/1 -> Sum4/2
  Demux3/2 -> To Workspace7/1
  Sum2/1 -> Scope5/1
  Demux4/2 -> Sum4/1
  Sum1/1 -> Mux1/1
  Demux4/1 -> Sum1/1
  Demux2/2 -> Sum3/1, To Workspace5/1, Scope4/2
  Mux1/1 -> Mux/3, Gain3/1
  Demux4/3 -> Sum5/1
  Constant/1 -> Sum2/2
  Rumore Additivo/1 -> Gain4/1
  Actuators/1(delta_F) -> Scope3/1, Mux2/1
  r_alfa/1 -> Mux/1
  r_beta/1 -> Mux/2

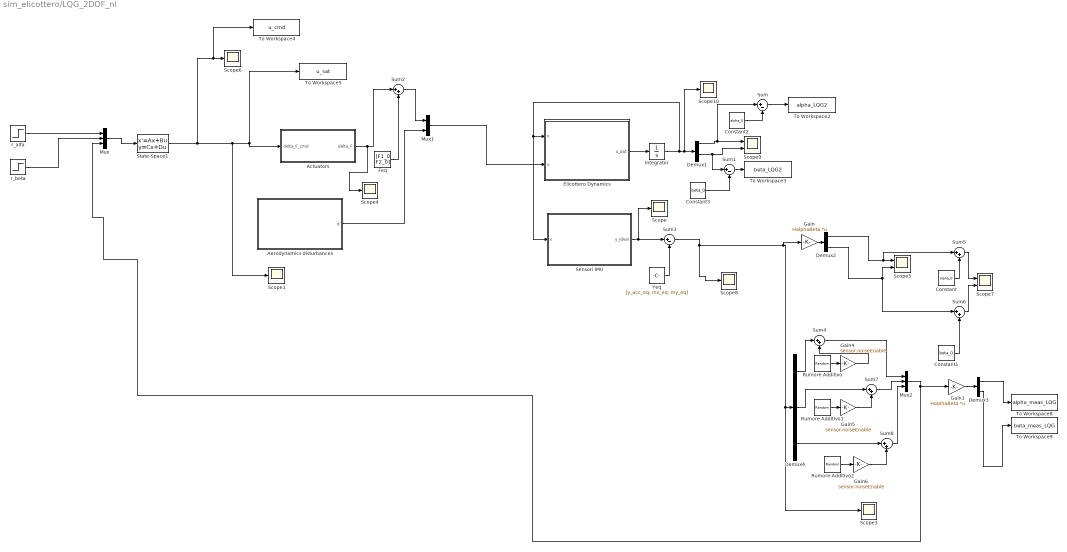
== system sim_elicottero/LQG_2DOF_nl ==
  Actuators : Subsystem
  Aerodynamics disturbances : Subsystem
  Constant : Constant  Value=alpha_0
  Constant1 : Constant  Value=beta_0
  Constant2 : Constant  Value=alpha_0
  Constant3 : Constant  Value=beta_0
  Demux1 : Demux
  Demux2 : Demux  Outputs=2
  Demux3 : Demux  Outputs=2
  Demux4 : Demux  Outputs=3
  Elicottero Dynamics : MATLAB Function  TreatAsAtomicUnit=on
  Feq : Constant  Value=[F1_0 F2_0]
  Gain : Gain  Gain=HalphaBeta  Multiplication=Matrix(K*u)
  Gain1 : Gain  Gain=HalphaBeta  Multiplication=Matrix(K*u)
  Gain4 : Gain  Gain=sensor.noiseEnable
  Gain5 : Gain  Gain=sensor.noiseEnable
  Gain6 : Gain  Gain=sensor.noiseEnable
  Integrator : Integrator  InitialCondition=[alpha_0; 0; beta_0; 0]
  Mux : Mux  Inputs=3
  Mux1 : Mux  Inputs=2
  Mux2 : Mux  Inputs=3
  Rumore Additivo : RandomNumber  Variance=sensor.acc.var  Seed=sensor.seed  SampleTime=sensor.acc.Ts
  Rumore Additivo1 : RandomNumber  Variance=sensor.mag.var  Seed=sensor.seed+1  SampleTime=sensor.mag.Ts
  Rumore Additivo2 : RandomNumber  Variance=sensor.mag.var  Seed=sensor.seed+2  SampleTime=sensor.mag.Ts
  Scope{,1,3..4,6,8,10} (7 alike) : Scope
      Scope settings: ActiveDisplayYMinimum=-1.6240661630355766  ActiveDisplayYMaximum=0.25200758348707814  DataLoggingVariableName=ScopeData22
      Scope1 settings: ActiveDisplayYMinimum=-0.85201275058268955  ActiveDisplayYMaximum=3.9243929593456111
      Scope10 settings: ActiveDisplayYMinimum=-0.021816615649929122  ActiveDisplayYMaximum=0.19634954084936207  DataLoggingVariableName=ScopeData24
      Scope3 settings: ActiveDisplayYMinimum=-1.6240661630355766  ActiveDisplayYMaximum=0.25200758348707814
      Scope4 settings: ActiveDisplayYMinimum=-0.11442663629112786  ActiveDisplayYMaximum=0.10867739086166754  DataLoggingVariableName=ScopeData4
      Scope6 settings: ActiveDisplayYMinimum=-1  ActiveDisplayYMaximum=1  DataLoggingVariableName=ScopeData6
      Scope8 settings: DataLoggingVariableName=ScopeData25
  Scope5 : Scope  NumInputPorts=2
      settings: ActiveDisplayYMinimum=-0.071940500775248273  ActiveDisplayYMaximum=0.07232150262419626  DataLoggingVariableName=ScopeData2
  Scope7 : Scope  NumInputPorts=2
      settings: ActiveDisplayYMinimum=-0.054900665423773753  ActiveDisplayYMaximum=0.26435366002895794  DataLoggingVariableName=ScopeData32
  Scope9 : Scope  NumInputPorts=2
      settings: ActiveDisplayYMinimum=-0.056861495742625029  ActiveDisplayYMaximum=0.28133520253821959  DataLoggingVariableName=ScopeData39
  Sensori IMU : MATLAB Function  TreatAsAtomicUnit=on
  State-Space1 : StateSpace  A=K_lqg_2dof.A  B=K_lqg_2dof.B  C=K_lqg_2dof.C  D=K_lqg_2dof.D  InitialCondition=0  ContinuousStateAttributes='stati_stimati'
  Sum : Sum  Inputs=|+-
  Sum1 : Sum  Inputs=|+-
  Sum{2,4..8} (6 alike) : Sum  Inputs=|++
  Sum3 : Sum  Inputs=|+-
  To Workspace2 : ToWorkspace  VariableName=alpha_LQG2  SaveFormat=Timeseries  SampleTime=-1
  To Workspace3 : ToWorkspace  VariableName=beta_LQG2  SaveFormat=Timeseries  SampleTime=-1
  To Workspace4 : ToWorkspace  VariableName=u_cmd  SaveFormat=Timeseries  SampleTime=-1
  To Workspace5 : ToWorkspace  VariableName=u_sat  SaveFormat=Timeseries  SampleTime=-1
  To Workspace8 : ToWorkspace  VariableName=alpha_meas_LQG  SaveFormat=Timeseries  SampleTime=-1
  To Workspace9 : ToWorkspace  VariableName=beta_meas_LQG  SaveFormat=Timeseries  SampleTime=-1
  Yeq : Constant  Value=[y_acc_eq; mx_eq; my_eq]
  r_alfa : Step  After=deg2rad(3)  SampleTime=0
  r_beta : Step  After=0  SampleTime=0
  wires:
  Mux/1 -> State-Space1/1
  Aerodynamics disturbances/1(d) -> Mux1/2
  Mux1/1 -> Elicottero Dynamics/2(u)
  Yeq/1 -> Sum3/2
  Integrator/1 -> Scope10/1, Demux1/1, Sensori IMU/1(x), Elicottero Dynamics/1(x)
  Sensori IMU/1(y_ideal) -> Sum3/1, Scope/1
  State-Space1/1 -> Actuators/1(delta_F_cmd), To Workspace5/1, Scope1/1, To Workspace4/1, Scope6/1
  Actuators/1(delta_F) -> Sum2/1, Scope4/1
  Sum4/1 -> Mux2/1
  Mux2/1 -> Mux/3, Gain1/1
  Gain4/1 -> Sum4/2
  Gain5/1 -> Sum7/2
  Demux2/1 -> Sum5/1, Scope5/1
  Sum3/1 -> Demux4/1, Scope3/1, Gain/1, Scope8/1
  Demux2/2 -> Sum6/1, Scope5/2
  Sum7/1 -> Mux2/2
  Demux4/3 -> Sum8/1
  Gain1/1 -> Demux3/1
  Rumore Additivo2/1 -> Gain6/1
  Demux4/1 -> Sum4/1
  Demux3/1 -> To Workspace8/1
  Demux3/2 -> To Workspace9/1
  Sum6/1 -> Scope7/2
  Gain/1 -> Demux2/1
  Rumore Additivo1/1 -> Gain5/1
  Demux4/2 -> Sum7/1
  Constant1/1 -> Sum6/2
  Rumore Additivo/1 -> Gain4/1
  Gain6/1 -> Sum8/2
  Sum8/1 -> Mux2/3
  Sum5/1 -> Scope7/1
  Constant/1 -> Sum5/2
  Feq/1 -> Sum2/2
  Sum2/1 -> Mux1/1
  Elicottero Dynamics/1(x_dot) -> Integrator/1
  r_alfa/1 -> Mux/1
  r_beta/1 -> Mux/2
  Sum/1 -> To Workspace2/1
  Demux1/1 -> Sum/1, Scope9/1
  Demux1/3 -> Sum1/1, Scope9/2
  Constant3/1 -> Sum1/2
  Sum1/1 -> To Workspace3/1
  Constant2/1 -> Sum/2

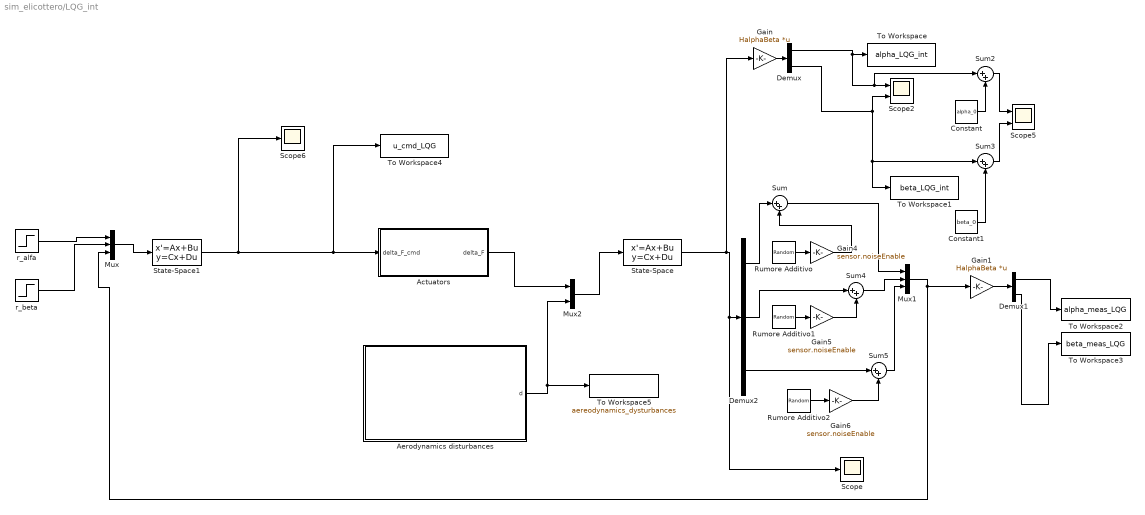
== system sim_elicottero/LQG_int ==
  Actuators : Subsystem
  Aerodynamics disturbances : Subsystem
  Constant : Constant  Value=alpha_0
  Constant1 : Constant  Value=beta_0
  Demux : Demux  Outputs=2
  Demux1 : Demux  Outputs=2
  Demux2 : Demux  Outputs=3
  Gain : Gain  Gain=HalphaBeta  Multiplication=Matrix(K*u)
  Gain1 : Gain  Gain=HalphaBeta  Multiplication=Matrix(K*u)
  Gain4 : Gain  Gain=sensor.noiseEnable
  Gain5 : Gain  Gain=sensor.noiseEnable
  Gain6 : Gain  Gain=sensor.noiseEnable
  Mux : Mux  Inputs=3
  Mux1 : Mux  Inputs=3
  Mux2 : Mux  Inputs=2
  Rumore Additivo : RandomNumber  Variance=sensor.acc.var  Seed=sensor.seed  SampleTime=sensor.acc.Ts
  Rumore Additivo1 : RandomNumber  Variance=sensor.mag.var  Seed=sensor.seed+1  SampleTime=sensor.mag.Ts
  Rumore Additivo2 : RandomNumber  Variance=sensor.mag.var  Seed=sensor.seed+2  SampleTime=sensor.mag.Ts
  Scope : Scope
      settings: ActiveDisplayYMinimum=-1.6240661630355766  ActiveDisplayYMaximum=0.25200758348707814  DataLoggingVariableName=ScopeData14
  Scope2 : Scope  NumInputPorts=2
      settings: ActiveDisplayYMinimum=-0.037068601532072296  ActiveDisplayYMaximum=0.10495677871134765  DataLoggingVariableName=ScopeData16
  Scope5 : Scope  NumInputPorts=2
      settings: ActiveDisplayYMinimum=-0.056599950333026186  ActiveDisplayYMaximum=0.28073891791993266  DataLoggingVariableName=ScopeData21
  Scope6 : Scope
      settings: ActiveDisplayYMinimum=-1  ActiveDisplayYMaximum=1  DataLoggingVariableName=ScopeData19
  State-Space : StateSpace  A=P_nom_ext.A  B=P_nom_ext.B  C=P_nom_ext.C  D=P_nom_ext.D  InitialCondition=0
  State-Space1 : StateSpace  A=K_lqg_int.A  B=K_lqg_int.B  C=K_lqg_int.C  D=K_lqg_int.D  InitialCondition=0  ContinuousStateAttributes='stati_stimati'
  Sum{,2..5} (5 alike) : Sum  Inputs=|++
  To Workspace : ToWorkspace  VariableName=alpha_LQG_int  SaveFormat=Timeseries  SampleTime=-1
  To Workspace1 : ToWorkspace  VariableName=beta_LQG_int  SaveFormat=Timeseries  SampleTime=-1
  To Workspace2 : ToWorkspace  VariableName=alpha_meas_LQG  SaveFormat=Timeseries  SampleTime=-1
  To Workspace3 : ToWorkspace  VariableName=beta_meas_LQG  SaveFormat=Timeseries  SampleTime=-1
  To Workspace4 : ToWorkspace  VariableName=u_cmd_LQG  SaveFormat=Timeseries  SampleTime=-1
  To Workspace5 : ToWorkspace  VariableName=aereodynamics_dysturbances  SaveFormat=Timeseries  SampleTime=-1
  r_alfa : Step  After=deg2rad(3)  SampleTime=0
  r_beta : Step  After=0  SampleTime=0
  wires:
  State-Space1/1 -> To Workspace4/1, Actuators/1(delta_F_cmd), Scope6/1
  Mux1/1 -> Gain1/1, Mux/3
  r_alfa/1 -> Mux/1
  Mux/1 -> State-Space1/1
  State-Space/1 -> Gain/1, Demux2/1, Scope/1
  r_beta/1 -> Mux/2
  Demux/1 -> Sum2/1, Scope2/1, To Workspace/1
  Demux/2 -> Sum3/1, To Workspace1/1, Scope2/2
  Constant/1 -> Sum2/2
  Sum2/1 -> Scope5/1
  Constant1/1 -> Sum3/2
  Sum3/1 -> Scope5/2
  Actuators/1(delta_F) -> Mux2/1
  Aerodynamics disturbances/1(d) -> To Workspace5/1, Mux2/2
  Mux2/1 -> State-Space/1
  Gain4/1 -> Sum/2
  Rumore Additivo/1 -> Gain4/1
  Demux2/1 -> Sum/1
  Rumore Additivo1/1 -> Gain5/1
  Demux2/2 -> Sum4/1
  Gain5/1 -> Sum4/2
  Sum4/1 -> Mux1/2
  Rumore Additivo2/1 -> Gain6/1
  Demux2/3 -> Sum5/1
  Gain6/1 -> Sum5/2
  Demux1/2 -> To Workspace3/1
  Demux1/1 -> To Workspace2/1
  Sum5/1 -> Mux1/3
  Sum/1 -> Mux1/1
  Gain/1 -> Demux/1
  Gain1/1 -> Demux1/1

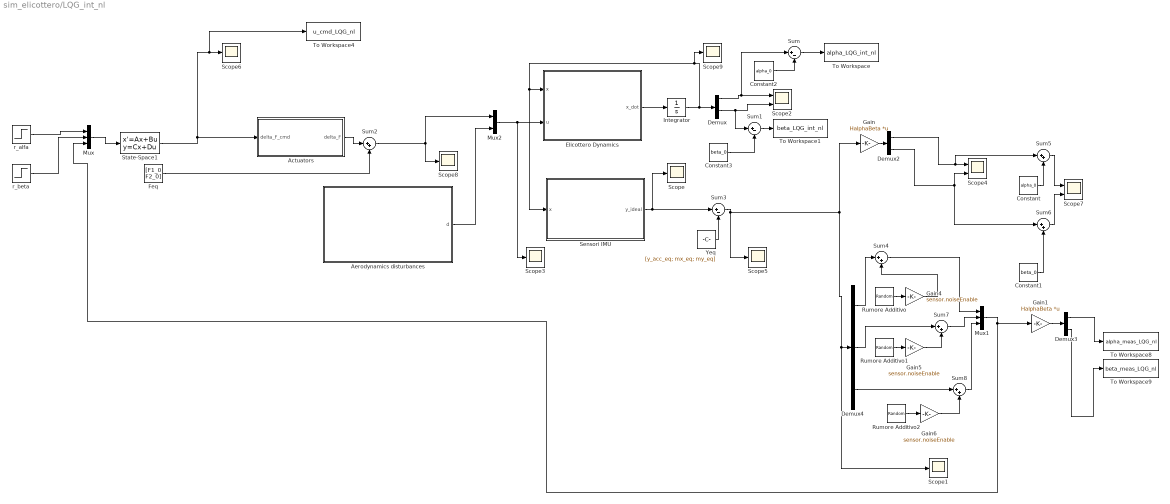
== system sim_elicottero/LQG_int_nl ==
  Actuators : Subsystem
  Aerodynamics disturbances : Subsystem
  Constant : Constant  Value=alpha_0
  Constant1 : Constant  Value=beta_0
  Constant2 : Constant  Value=alpha_0
  Constant3 : Constant  Value=beta_0
  Demux : Demux
  Demux2 : Demux  Outputs=2
  Demux3 : Demux  Outputs=2
  Demux4 : Demux  Outputs=3
  Elicottero Dynamics : MATLAB Function  TreatAsAtomicUnit=on
  Feq : Constant  Value=[F1_0 F2_0]
  Gain : Gain  Gain=HalphaBeta  Multiplication=Matrix(K*u)
  Gain1 : Gain  Gain=HalphaBeta  Multiplication=Matrix(K*u)
  Gain4 : Gain  Gain=sensor.noiseEnable
  Gain5 : Gain  Gain=sensor.noiseEnable
  Gain6 : Gain  Gain=sensor.noiseEnable
  Integrator : Integrator  InitialCondition=[alpha_0; 0; beta_0; 0]
  Mux : Mux  Inputs=3
  Mux1 : Mux  Inputs=3
  Mux2 : Mux  Inputs=2
  Rumore Additivo : RandomNumber  Variance=sensor.acc.var  Seed=sensor.seed  SampleTime=sensor.acc.Ts
  Rumore Additivo1 : RandomNumber  Variance=sensor.mag.var  Seed=sensor.seed+1  SampleTime=sensor.mag.Ts
  Rumore Additivo2 : RandomNumber  Variance=sensor.mag.var  Seed=sensor.seed+2  SampleTime=sensor.mag.Ts
  Scope{,1,3,5..6,8..9} (7 alike) : Scope
      Scope settings: ActiveDisplayYMinimum=-2.6695864737629402  ActiveDisplayYMaximum=1.4000873242913907  DataLoggingVariableName=ScopeData14
      Scope1 settings: ActiveDisplayYMinimum=-1.6240661630355766  ActiveDisplayYMaximum=0.25200758348707814  DataLoggingVariableName=ScopeData15
      Scope3 settings: ActiveDisplayYMinimum=-0.066808898460173932  ActiveDisplayYMaximum=0.16260152032849579  DataLoggingVariableName=ScopeData17
      Scope5 settings: ActiveDisplayYMinimum=-0.69850075039123272  ActiveDisplayYMaximum=0.69520204307189137  DataLoggingVariableName=ScopeData20
      Scope6 settings: ActiveDisplayYMinimum=-0.13657354328857155  ActiveDisplayYMaximum=0.3937278655924531  DataLoggingVariableName=ScopeData19
      Scope8 settings: ActiveDisplayYMinimum=-0.16116164249761136  ActiveDisplayYMaximum=0.54820504636646727  DataLoggingVariableName=ScopeData27
      Scope9 settings: ActiveDisplayYMinimum=-0.021816615649929122  ActiveDisplayYMaximum=0.19634954084936207  DataLoggingVariableName=ScopeData28
  Scope2 : Scope  NumInputPorts=2
      settings: ActiveDisplayYMinimum=-0.056861495742625029  ActiveDisplayYMaximum=0.28133520253821959  DataLoggingVariableName=ScopeData16
  Scope4 : Scope  NumInputPorts=2
      settings: ActiveDisplayYMinimum=-0.033068887345671219  ActiveDisplayYMaximum=0.0678695412426075  DataLoggingVariableName=ScopeData18
  Scope7 : Scope  NumInputPorts=2
      settings: ActiveDisplayYMinimum=-0.054885502995600327  ActiveDisplayYMaximum=0.26421908209196954  DataLoggingVariableName=ScopeData26
  Sensori IMU : MATLAB Function  TreatAsAtomicUnit=on
  State-Space1 : StateSpace  A=K_lqg_int.A  B=K_lqg_int.B  C=K_lqg_int.C  D=K_lqg_int.D  InitialCondition=0  ContinuousStateAttributes='stati_stimati'
  Sum : Sum  Inputs=|+-
  Sum1 : Sum  Inputs=|+-
  Sum{2,4..8} (6 alike) : Sum  Inputs=|++
  Sum3 : Sum  Inputs=|+-
  To Workspace : ToWorkspace  VariableName=alpha_LQG_int_nl  SaveFormat=Timeseries  SampleTime=-1
  To Workspace1 : ToWorkspace  VariableName=beta_LQG_int_nl  SaveFormat=Timeseries  SampleTime=-1
  To Workspace4 : ToWorkspace  VariableName=u_cmd_LQG_nl  SaveFormat=Timeseries  SampleTime=-1
  To Workspace8 : ToWorkspace  VariableName=alpha_meas_LQG_nl  SaveFormat=Timeseries  SampleTime=-1
  To Workspace9 : ToWorkspace  VariableName=beta_meas_LQG_nl  SaveFormat=Timeseries  SampleTime=-1
  Yeq : Constant  Value=[y_acc_eq; mx_eq; my_eq]
  r_alfa : Step  After=deg2rad(3)  SampleTime=0
  r_beta : Step  After=0  SampleTime=0
  wires:
  r_alfa/1 -> Mux/1
  State-Space1/1 -> Actuators/1(delta_F_cmd), To Workspace4/1, Scope6/1
  Mux2/1 -> Scope3/1, Elicottero Dynamics/2(u)
  Mux/1 -> State-Space1/1
  Aerodynamics disturbances/1(d) -> Mux2/2
  r_beta/1 -> Mux/2
  Demux/1 -> Sum/1, Scope2/1
  Demux/3 -> Sum1/1, Scope2/2
  Elicottero Dynamics/1(x_dot) -> Integrator/1
  Integrator/1 -> Scope9/1, Sensori IMU/1(x), Elicottero Dynamics/1(x), Demux/1
  Feq/1 -> Sum2/2
  Sensori IMU/1(y_ideal) -> Sum3/1, Scope/1
  Yeq/1 -> Sum3/2
  Sum7/1 -> Mux1/2
  Constant1/1 -> Sum6/2
  Sum8/1 -> Mux1/3
  Demux4/1 -> Sum4/1
  Rumore Additivo/1 -> Gain4/1
  Gain6/1 -> Sum8/2
  Sum6/1 -> Scope7/2
  Rumore Additivo2/1 -> Gain6/1
  Demux3/2 -> To Workspace9/1
  Rumore Additivo1/1 -> Gain5/1
  Gain5/1 -> Sum7/2
  Demux3/1 -> To Workspace8/1
  Sum4/1 -> Mux1/1
  Demux4/3 -> Sum8/1
  Constant/1 -> Sum5/2
  Demux2/2 -> Sum6/1, Scope4/2
  Gain1/1 -> Demux3/1
  Demux4/2 -> Sum7/1
  Demux2/1 -> Sum5/1, Scope4/1
  Gain/1 -> Demux2/1
  Sum3/1 -> Demux4/1, Scope1/1, Gain/1, Scope5/1
  Gain4/1 -> Sum4/2
  Sum5/1 -> Scope7/1
  Mux1/1 -> Mux/3, Gain1/1
  Actuators/1(delta_F) -> Sum2/1
  Sum2/1 -> Scope8/1, Mux2/1
  Constant2/1 -> Sum/2
  Sum/1 -> To Workspace/1
  Sum1/1 -> To Workspace1/1
  Constant3/1 -> Sum1/2

== system sim_elicottero/Verifica Dinamica ==
  Constant : Constant  Value=0
  Constant1 : Constant  Value=[0 0]
  Constant2 : Constant  Value=0
  Constant3 : Constant  Value=2
  Elicottero Dynamics : MATLAB Function  TreatAsAtomicUnit=on
  Feq : Constant  Value=[F1_0 F2_0]
  Integrator : Integrator  InitialCondition=[alpha_0; 0; beta_0; 0]
  Multiport Switch : MultiPortSwitch  SaturateOnIntegerOverflow=off  InputSameDT=off
  Mux : Mux  Inputs=2
  Mux1 : Mux  Inputs=2
  Scope : Scope
      settings: ActiveDisplayYMinimum=-0.0886741790010199  ActiveDisplayYMaximum=0.49466636766520478  DataLoggingVariableName=ScopeData43
  Scope1 : Scope
      settings: ActiveDisplayYMinimum=-1  ActiveDisplayYMaximum=1  DataLoggingVariableName=ScopeData44
  Scope2 : Scope
      settings: ActiveDisplayYMinimum=-0.013087539672587651  ActiveDisplayYMaximum=0.022905294586664859  DataLoggingVariableName=ScopeData45
  Step : Step  After=0.03407  SampleTime=0
  Step1 : Step  After=0.00060074  SampleTime=0
  Sum : Sum  Inputs=|++
  wires:
  Elicottero Dynamics/1(x_dot) -> Integrator/1
  Step/1 -> Mux/1
  Mux/1 -> Multiport Switch/2
  Multiport Switch/1 -> Sum/1, Scope1/1
  Constant/1 -> Mux/2
  Constant1/1 -> Multiport Switch/3
  Feq/1 -> Sum/2
  Sum/1 -> Scope2/1, Elicottero Dynamics/2(u)
  Integrator/1 -> Elicottero Dynamics/1(x), Scope/1
  Constant2/1 -> Mux1/1
  Step1/1 -> Mux1/2
  Mux1/1 -> Multiport Switch/4
  Constant3/1 -> Multiport Switch/1

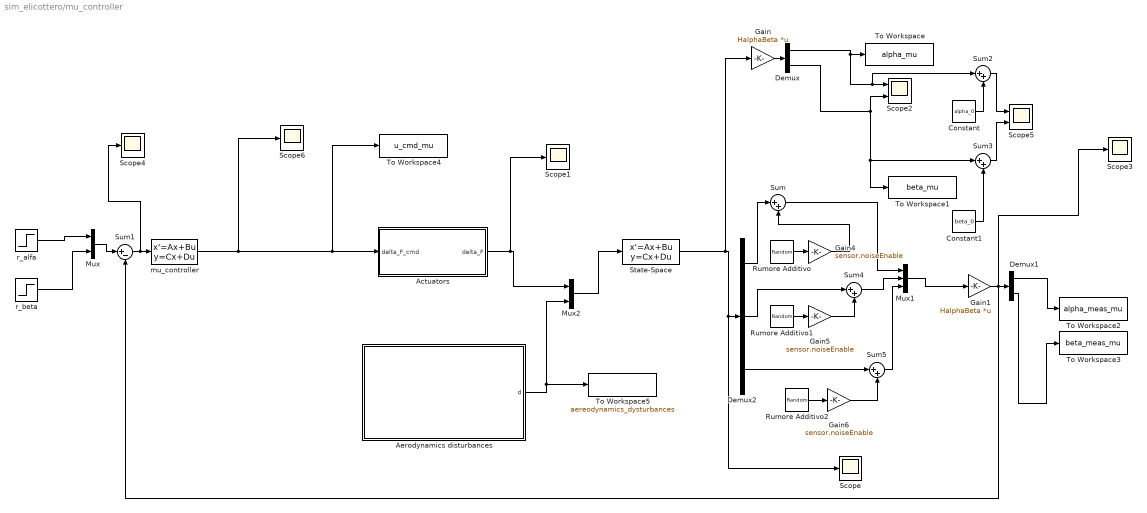
== system sim_elicottero/mu_controller ==
  Actuators : Subsystem
  Aerodynamics disturbances : Subsystem
  Constant : Constant  Value=alpha_0
  Constant1 : Constant  Value=beta_0
  Demux : Demux  Outputs=2
  Demux1 : Demux  Outputs=2
  Demux2 : Demux  Outputs=3
  Gain : Gain  Gain=HalphaBeta  Multiplication=Matrix(K*u)
  Gain1 : Gain  Gain=HalphaBeta  Multiplication=Matrix(K*u)
  Gain4 : Gain  Gain=sensor.noiseEnable
  Gain5 : Gain  Gain=sensor.noiseEnable
  Gain6 : Gain  Gain=sensor.noiseEnable
  Mux : Mux  Inputs=2
  Mux1 : Mux  Inputs=3
  Mux2 : Mux  Inputs=2
  Rumore Additivo : RandomNumber  Variance=sensor.acc.var  Seed=sensor.seed  SampleTime=sensor.acc.Ts
  Rumore Additivo1 : RandomNumber  Variance=sensor.mag.var  Seed=sensor.seed+1  SampleTime=sensor.mag.Ts
  Rumore Additivo2 : RandomNumber  Variance=sensor.mag.var  Seed=sensor.seed+2  SampleTime=sensor.mag.Ts
  Scope{,1,3..4,6} (5 alike) : Scope
      Scope settings: ActiveDisplayYMinimum=-1.6240661630355766  ActiveDisplayYMaximum=0.25200758348707814  DataLoggingVariableName=ScopeData14
      Scope1 settings: ActiveDisplayYMinimum=-0.31965763186145552  ActiveDisplayYMaximum=0.334460216852247  DataLoggingVariableName=ScopeData23
      Scope3 settings: DataLoggingVariableName=ScopeData36
      Scope4 settings: ActiveDisplayYMinimum=-0.42095947729345456  ActiveDisplayYMaximum=0.43773263079957025  DataLoggingVariableName=ScopeData42
      Scope6 settings: ActiveDisplayYMinimum=-0.47606356951282441  ActiveDisplayYMaximum=0.525266126912983  DataLoggingVariableName=ScopeData19
  Scope2 : Scope  NumInputPorts=2
      settings: ActiveDisplayYMinimum=-0.070504242439614381  ActiveDisplayYMaximum=0.10697690957361014  DataLoggingVariableName=ScopeData16
  Scope5 : Scope  NumInputPorts=2
      settings: ActiveDisplayYMinimum=-0.072362132475087784  ActiveDisplayYMaximum=0.2803562626809285  DataLoggingVariableName=ScopeData21
  State-Space : StateSpace  A=P_nom_ext.A  B=P_nom_ext.B  C=P_nom_ext.C  D=P_nom_ext.D  InitialCondition=0
  Sum{,2..5} (5 alike) : Sum  Inputs=|++
  Sum1 : Sum  Inputs=|+-
  To Workspace : ToWorkspace  VariableName=alpha_mu  SaveFormat=Timeseries  SampleTime=-1
  To Workspace1 : ToWorkspace  VariableName=beta_mu  SaveFormat=Timeseries  SampleTime=-1
  To Workspace2 : ToWorkspace  VariableName=alpha_meas_mu  SaveFormat=Timeseries  SampleTime=-1
  To Workspace3 : ToWorkspace  VariableName=beta_meas_mu  SaveFormat=Timeseries  SampleTime=-1
  To Workspace4 : ToWorkspace  VariableName=u_cmd_mu  SaveFormat=Timeseries  SampleTime=-1
  To Workspace5 : ToWorkspace  VariableName=aereodynamics_dysturbances  SaveFormat=Timeseries  SampleTime=-1
  mu_controller : StateSpace  A=K_mu.A  B=K_mu.B  C=K_mu.C  D=K_mu.D  InitialCondition=zeros(size(K_mu.A,1),1)
  r_alfa : Step  After=deg2rad(3)  SampleTime=0
  r_beta : Step  After=0  SampleTime=0
  wires:
  mu_controller/1 -> To Workspace4/1, Actuators/1(delta_F_cmd), Scope6/1
  Mux1/1 -> Gain1/1
  r_alfa/1 -> Mux/1
  Mux/1 -> Sum1/1
  State-Space/1 -> Gain/1, Demux2/1, Scope/1
  r_beta/1 -> Mux/2
  Demux/1 -> Sum2/1, Scope2/1, To Workspace/1
  Demux/2 -> Sum3/1, To Workspace1/1, Scope2/2
  Constant/1 -> Sum2/2
  Sum2/1 -> Scope5/1
  Constant1/1 -> Sum3/2
  Sum3/1 -> Scope5/2
  Actuators/1(delta_F) -> Scope1/1, Mux2/1
  Aerodynamics disturbances/1(d) -> To Workspace5/1, Mux2/2
  Mux2/1 -> State-Space/1
  Gain4/1 -> Sum/2
  Rumore Additivo/1 -> Gain4/1
  Demux2/1 -> Sum/1
  Rumore Additivo1/1 -> Gain5/1
  Demux2/2 -> Sum4/1
  Gain5/1 -> Sum4/2
  Sum4/1 -> Mux1/2
  Rumore Additivo2/1 -> Gain6/1
  Demux2/3 -> Sum5/1
  Gain6/1 -> Sum5/2
  Demux1/2 -> To Workspace3/1
  Demux1/1 -> To Workspace2/1
  Sum5/1 -> Mux1/3
  Sum/1 -> Mux1/1
  Gain/1 -> Demux/1
  Gain1/1 -> Scope3/1, Demux1/1, Sum1/2
  Sum1/1 -> Scope4/1, mu_controller/1
